simulink model "Assignment2a"  (R2022a)
settings: Solver=FixedStepAuto  StartTime=0.0  StopTime=inf  FixedStep=0.01  RelTol=1e-3
values from neighbouring files (symbols this model uses):
  WaypointList = [ 5,  0, pi/2 ... (first row only)    [A1_ScriptForWPMatrix.m]
undefined symbols (not defined in the file or in its folder): Angular, index, Linear
libraries: robotlib x3, simulink x1, dspindex x1
settings Model: Creator=jacopo  LastModifiedBy=jacopo
settings OptimizationCC: EnhancedBackFolding=on  PassReuseOutputArgsAs=Individual arguments  ZeroExternalMemoryAtStartup=off  ZeroInternalMemoryAtStartup=off  MaxStackSize=64  OptimizeBlockOrder=speed  DifferentSizesBufferReuse=on  OptimizationCustomize=off  EfficientTunableParamExpr=on
settings DebuggingCC: ParameterTunabilityLossMsg=error
settings HardwareCC: ProdBitPerPointer=32  ProdBitPerSizeT=32  ProdBitPerPtrDiffT=32  ProdLargestAtomicFloat=None  ProdIntDivRoundTo=Undefined  ProdEndianess=Unspecified  ProdWordSize=32  ProdHWDeviceType=Generic->Unspecified (assume 32-bit Generic)
settings SFSimCC: MATLABDynamicMemAlloc=off
settings RTWCC: SystemTargetFile=ert.tlc  HardwareBoard=Robot Operating System (ROS)  TLCOptions="-aInlineSetEventsForThisBaseRateFcn=TLC_FALSE -aSuppressMultiTaskScheduler=TLC_FALSE  -aRateBasedStepFcn=0"  TemplateMakefile=ert_default_tmf  Toolchain=Catkin  TargetLang=C++
settings CodeAppCC: ForceParamTrailComments=on  IgnoreCustomStorageClasses=off  OperatorAnnotations=on  SimulinkDataObjDesc=on  SFDataObjDesc=on  InsertBlockDesc=on

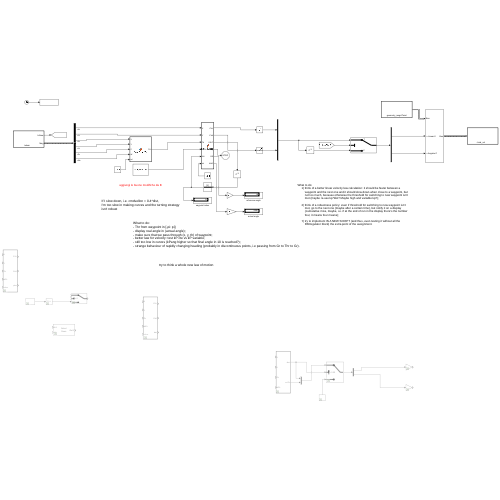
[thumbnail: Simulink's stored preview of the top-level diagram]
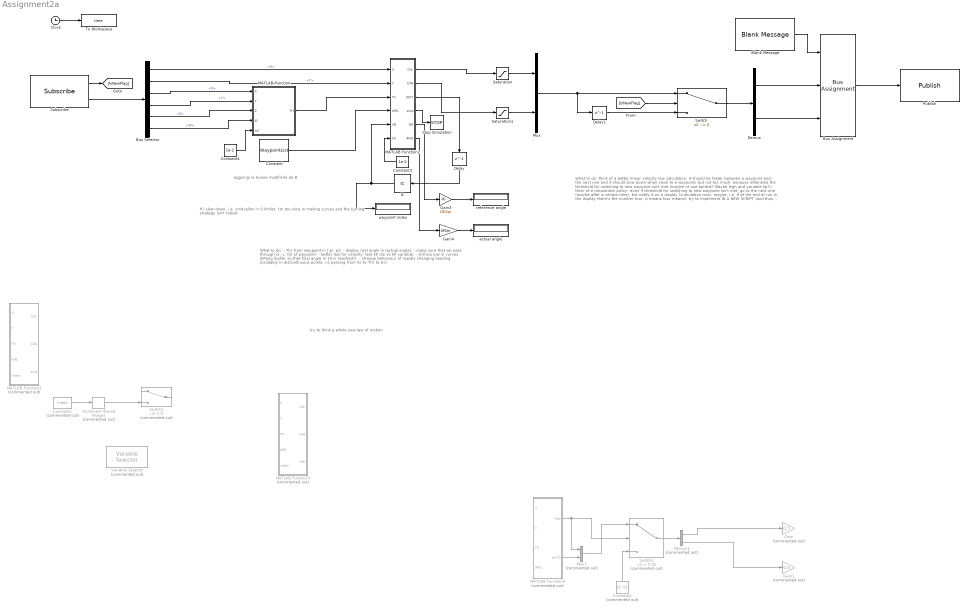
== system Assignment2a ==
  note: aggiungi le buone modifiche da B
  note: try to think a whole new law of motion
  note: If I slow down, i.e. cmdvellon = 0.4*dist,
      | I'm too slow in making curves and the turning strategy
      | isn't robust
  note: What to do:
      | - Thr from waypoint in [-pi: pi];
      | - display real angle in (actual angle);
      | - make sure that we pass through (x, y, th) of waypoint;
      | - better law for velocity: test kP cte vs kP variable;
      | - still too low in curves (kPang higher so that final angle in 10 is reached?);
      | - strange behaviour of rapidly changing heading (probably in discontinuous points, i.e passing from Gr to Thr to Gr).
  note: What to do:
      | think of a better linear velocity law calculation: it should be faster between a waypoint and the next one and it should slow down when close to a waypoint, but not too much, because otherwise the threshold for switching to new waypoint isn't met (maybe re-use kp*dist? Maybe high and variable kp?);
      |
      | think of a robustness policy: even if threshold for switching to new waypoint isn't met, go to the next one (maybe after a certain time), but notify it on a display (cumulative miss, maybe, i.e. if at the end of run in the display there's the number four, it means four means);
      |
      | try to implement IN A NEW SCRIPT (and thus, even testing it without all the FBRegulator block) the extra point of the assignment.
  Blank Message : robotlib/Blank Message  messageClass=Message  entityType=geometry_msgs/Twist  messageType=geometry_msgs/Twist  SampleTime=inf  legacyBusStruct=off
  Bus Assignment : BusAssignment  AssignedSignals=Linear.X,Angular.Z
  Bus Selector : BusSelector  OutputSignals=Pose.Pose.Position.X,Pose.Pose.Position.Y,Pose.Pose.Orientation.X,Pose.Pose.Orientation.Y,Pose.Pose.Orientation.Z,Pose.Pose.Orientation.W
  Clock : Clock
  Constant : Constant  Value=WaypointList
  Constant1 : Constant  Commented=on  Value=index
  Constant2 : Constant  Commented=on  Value=[0; 0]
  Constant3 : Constant  Value=1e-2
  Constant4 : Constant  Value=1e-2
  Delay : Delay  DelayLength=1
  Delay1 : Delay  DelayLength=1
  Demux : Demux  Outputs=2
  Demux1 : Demux  Commented=on  Outputs=2
  Gain : Gain  Commented=on  Gain=0.5
  Gain1 : Gain  Commented=on  Gain=0.5
  Gain3 : Gain  Gain=180/pi
  Gain4 : Gain  Gain=180/pi
  IC : InitialCondition
  Increment Stored Integer : simulink/Additional Math & Discrete/Additional Math: Increment - Decrement/Increment Stored Integer  Commented=on
  MATLAB Function : MATLAB Function  TreatAsAtomicUnit=on
  MATLAB Function1 : MATLAB Function  Commented=on  TreatAsAtomicUnit=on
  MATLAB Function2 : MATLAB Function  TreatAsAtomicUnit=on
  MATLAB Function3 : MATLAB Function  Commented=on  TreatAsAtomicUnit=on
  MATLAB Function4 : MATLAB Function  Commented=on  TreatAsAtomicUnit=on
  Mux : Mux  Inputs=2
  Mux1 : Mux  Commented=on  Inputs=2
  Publish : robotlib/Publish  topicSource=Select from ROS network  topic=/cmd_vel  messageType=geometry_msgs/Twist  legacyBusStruct=off  messageQueueLength=1
  Saturation : Saturate  UpperLimit=0.2  LowerLimit=-0.2
  Saturation1 : Saturate  UpperLimit=0.4  LowerLimit=-0.4
  Stop Simulation : Stop
  Subscribe : robotlib/Subscribe  topicSource=Select from ROS network  topic=/odom  messageType=nav_msgs/Odometry  SampleTime=-1  legacyBusStruct=off  messageQueueLength=1
  Switch : Switch  Criteria=u2 ~= 0  SaturateOnIntegerOverflow=off  InputSameDT=off
  Switch1 : Switch  Commented=on  Criteria=u2 > Threshold  SaturateOnIntegerOverflow=off  InputSameDT=off
  Switch2 : Switch  Commented=on  Criteria=u2 > Threshold  Threshold=0.05  SaturateOnIntegerOverflow=off  InputSameDT=off
  To Workspace : ToWorkspace  VariableName=time  SampleTime=-1
  Variable Selector : dspindex/Variable Selector  Commented=on  NumInputs=1  rowsOrCols=Rows  IdxMode=Variable  Elements=[1 3]  ZerOneIdxMode=One-based  errmode=Clip Index  FillMode=on  FillValues=0
  actual angle : Display
  reference angle : Display
  waypoint index : Display
  wires:
  Subscribe/2 -> Bus Selector/1
  Bus Selector/3 -> MATLAB Function/1(X)  "<X>"
  Bus Selector/4 -> MATLAB Function/2(Y)  "<Y>"
  Bus Selector/5 -> MATLAB Function/3(Z)  "<Z>"
  Bus Selector/6 -> MATLAB Function/4(W)  "<W>"
  Constant/1 -> MATLAB Function2/4(WPL)
  MATLAB Function/1(TH) -> MATLAB Function2/3(Th)
  Bus Selector/2 -> MATLAB Function2/2(Y)  "<Y>"
  Bus Selector/1 -> MATLAB Function2/1(X)  "<X>"
  MATLAB Function2/1(CVL) -> Saturation/1
  MATLAB Function2/2(CVA) -> Saturation1/1
  Subscribe/1 -> [IsNewFlag]
  [IsNewFlag] -> Switch/2
  Saturation/1 -> Mux/1
  Saturation1/1 -> Mux/2
  Mux/1 -> Delay1/1, Switch/1
  Switch/1 -> Demux/1
  Blank Message/1 -> Bus Assignment/1
  Demux/1 -> Bus Assignment/2
  Demux/2 -> Bus Assignment/3
  Bus Assignment/1 -> Publish/1
  Clock/1 -> To Workspace/1
  Constant1/1 -> Increment Stored Integer/1
  Increment Stored Integer/1 -> Switch1/3
  Switch2/1 -> Demux1/1
  MATLAB Function4/1(dist) -> Mux1/1, Switch2/2
  Constant2/1 -> Switch2/3
  Demux1/2 -> Gain1/1
  MATLAB Function4/2(errTh) -> Mux1/2
  Demux1/1 -> Gain/1
  Mux1/1 -> Switch2/1
  IC/1 -> waypoint index/1, MATLAB Function2/5(IIN)
  Delay/1 -> IC/1
  MATLAB Function2/3(IOUT) -> Delay/1
  MATLAB Function2/4(stop) -> Stop Simulation/1
  Delay1/1 -> Switch/3
  Constant3/1 -> MATLAB Function2/6(tol)
  MATLAB Function2/5(GR) -> Gain3/1
  Gain3/1 -> reference angle/1
  Gain4/1 -> actual angle/1
  Constant4/1 -> MATLAB Function/5(tol)
  MATLAB Function2/6(ANG) -> Gain4/1

== matlab function Assignment2a/MATLAB Function1 ==
  data: X input; CVL output; Y input; Th input; WPL input; CVA output; index input; plus output
function [CVL, CVA, plus] = FBRegulator(X, Y, Th, WPL, index)

kP = 0.5;

POSd = WPL(index,:);

Xd = POSd(1); Yd = POSd(2); Thd = POSd(3);

% errX  = X - Xd;
% errY  = Y - Yd;

dist = sqrt( (X - Xd)^2 + (Y - Yd)^2 );
errTh = Th - Thd;

CVL = kP*dist;
CVA = kP*errTh;

if dist <= 0.05
    if index == 10    
        CVL = 0;
        CVA = 0;
    end
%    plus = index + 1;
   plus = 1;
end

== matlab function Assignment2a/MATLAB Function ==
  data: X input; TH output; Y input; Z input; W input; tol input
function TH = fromQuat2Eu(X, Y, Z, W, tol)



ANGLE = quat2eul([W, X, Y, Z]);

TH = ANGLE(1);

% following is mod

% if - pi + tol < TH && TH < - pi/2 - tol % TH < -tol
%     TH = TH + 2*pi;
% end

% not robust mod (ok 4 -> 5 and 5 -> 6, original problem returns for 7 -> 8 
%     if TH < - tol
%         if  ( TH + 2*pi ) > 300*pi/180
%             TH = TH;
%         else
%             TH = TH + 2*pi;
%         end
%     end

== matlab function Assignment2a/MATLAB Function2 ==
  data: X input; CVL output; Y input; Th input; WPL input; CVA output; IOUT output; IIN input; stop output; tol input; GR output; ANG output
function [CVL, CVA, IOUT, stop, GR, ANG] = FBRegulator(X, Y, Th, WPL, IIN, tol)

kPL = 1;
kPA = 1.4; %0.8 %1.2

POSr = WPL(IIN, :);

Xr = POSr(1); Yr = POSr(2); Thr = POSr(3);
if pi < Thr && Thr < 2*pi
    Thr = Thr - 2*pi;
end

Z = (Xr - X) + 1i*(Yr - Y);

% dist = sqrt( (Xr - X)^2 + (Yr - Y)^2 );
dist = abs(Z);

if dist <= 0.2
    kPL = 0.4;
end

if dist <= 0.1
    errTh = Thr - Th;
%     kPL = 0.4; % 0.6, % 0.2
    kPL = 0.2; % faster attempt: should we also modify tolerance on dist?
    GR = Thr; %debugging purposes
else
    % here there was ***
    Gr = angle(Z);

    if (Th > tol) && (- pi + tol < Gr && Gr < - pi/2 - tol) % Gr < - tol
%         if  ( Gr + 2*pi ) > 300*pi/180   %
%             Gr = Gr;                     %
%         else                             % solves 4->5, 5->6, but worsens 7->8
%             Gr = Gr + 2*pi;
%         end
        Gr = Gr + 2*pi;
    elseif (- pi + tol < Th && Th < - pi/2 - tol) && (Gr > tol)
        Th = Th + 2*pi;
    end

    errTh = Gr - Th;
    GR = Gr;
end

ANG = Th;

% CVL = kPL*dist;
% CVL = kPL*0.1;
% CVL = kPL*0.2; % faster attempt
CVL = 0.6*dist; %0.8 original, %0.4 not robust
CVA = kPA*errTh;


if dist <= 0.05 
   stop = 0;
   IOUT = IIN + 1;
   if IIN == 10 % probably this condition has to be switched somewhere else
       CVL = 0;
       CVA = 0;
       stop = 1;
   end
%    IOUT = IIN + 1;
else
    IOUT = IIN;
    stop = 0;
end


% following was *** original condition
%  %( real(Z) < 0 && imag(Z) < 0 ) || ( real(Z) > 0 && imag(Z) < 0 ) % it's better to use <-tol and >tol
%     if ( real(Z) < -tol && imag(Z) < -tol ) || ( real(Z) > tol && imag(Z) < -tol )
%         Gr = 2*pi - abs( angle(Z) ); %----> problem is here!
% %         Gr = angle(Z);
%     else
%         Gr = angle(Z);
%     end

== matlab function Assignment2a/MATLAB Function3 ==
  data: X input; CVL output; Y input; Th input; WPL input; CVA output; index input; dist output
function [CVL, CVA, dist] = FBRegulator(X, Y, Th, WPL, index)

kP = 0.5;

POSd = WPL(index, :); 

Xd = POSd(1); Yd = POSd(2); Thd = POSd(3);

% errX  = X - Xd;
% errY  = Y - Yd;

dist = sqrt( (X - Xd)^2 + (Y - Yd)^2 );
errTh = Th - Thd;

CVL = kP*dist;
CVA = kP*errTh;

if dist <= 0.05
    if index == 10    
        CVL = 0;
        CVA = 0;
    end
end

== matlab function Assignment2a/MATLAB Function4 ==
  data: X input; dist output; Y input; Th input; WPL input; errTh output
function [dist, errTh] = fcn(X, Y, Th, WPL)

Xr = WPL(1); Yr = WPL(2); Thr = WPL(3);

dist = sqrt( (Xr - X)^2 + (Yr - Y)^2 );

errT = Thr - Th;
end
